simulink library "WECSim_Lib"  (R2019b)
settings: Solver=ode45  StartTime=0.0  StopTime=10.0  RelTol=1e-3  EnableMultiTasking=on
undefined symbols (not defined in the file): body, constraint, mooring, pto, simu, waves, X, Y, Z
libraries: nesl_utility x124, sm_lib x101, $bdroot x14, vrlib x2
(part 1 of 9)
settings Model: Creator=cmichel  LastModifiedBy=ntom
settings DataIOCC: LimitDataPoints=on  SaveFormat=Array  SignalLoggingSaveFormat=ModelDataLogs  ReturnWorkspaceOutputs=off
settings OptimizationCC: LifeSpan=inf
settings DebuggingCC: UnderspecifiedInitializationDetection=Classic  MergeDetectMultiDrivingBlocksExec=none  SolverPrmCheckMsg=warning  MultiTaskDSMMsg=warning  MultiTaskCondExecSysMsg=none  AllowSymbolicDim=off  SFUnexpectedBacktrackingDiag=warning  SFNoUnconditionalDefaultTransitionDiag=warning  SFExecutionAtInitializationDiag=none  ArithmeticOperatorsInVariantConditions=warning
settings HardwareCC: ProdBitPerPointer=32  ProdBitPerSizeT=32  ProdBitPerPtrDiffT=32  ProdLargestAtomicFloat=None  ProdIntDivRoundTo=Undefined  ProdEndianess=Unspecified  ProdWordSize=32  ProdHWDeviceType=32-bit Generic
settings ModelReferenceCC: PropagateSignalLabelsOutOfModel=off
settings SFSimCC: SimUseLocalCustomCode=off  CustomCodeUndefinedFunction=UseInterfaceOnly
settings RTWCC: RTWUseLocalCustomCode=off
settings CodeAppCC: StateflowObjectComments=on
settings GRTTargetCC: TargetLangStandard=C89/C90 (ANSI)
settings ConfigComp: CovMetricSettings=dw  CovSaveCumulativeToWorkspaceVar=on  CovSaveSingleToWorkspaceVar=on  CovExternalEMLEnable=off  CovSFcnEnable=off

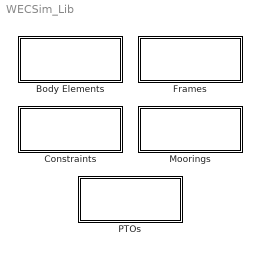
== system WECSim_Lib ==
  Body Elements : Subsystem
      mask Display: text(0,0,' ')
  Constraints : Subsystem
      mask Display: text(0,0,' ')
  Frames : Subsystem
      mask Display: text(0,0,' ')
  Moorings : Subsystem
      mask Display: text(0,0,' ')
  PTOs : Subsystem
      mask Display: text(0,0,' ')

== system WECSim_Lib/Body Elements ==
  Flex Body : Subsystem  VariantControl=(default)  mask(Flex Body){body=body(1), InputFileText=Global Reference Frame option "Use Input File" is selected., h5File=hydroData/*.h5, geometryFile=geometry/*.stl, mass=0, momOfInertia=0 0 0, nhBody=0, flexHydroBody=1, cg=0 0 0, cb=0 0 0, dof=, dispVol=0, initLinDisp=0 0 0, initAngularDispAxis=0 1 0, initAngularDispAngle=0, cd=0 0 0, ca=0 0 0, characteristicArea=0 0 0, VME=0, rgME=0 0 0, z=0 0 1}
      mask prompts: body "Body Number:"; mass "Body Mass [kg]:"; momOfInertia "MoI [kg*m^2]:"; nhBody "Non-hydro Body"; flexHydroBody "Flexible Body"; cg "Center of gravity [m]"; cb "Center of buoyancy [m]"; dof "Degrees of freedom"; dispVol "Displaced Volume [m^3]"; initLinDisp "Initial Linear Displacement"; initAngularDispAxis "Initial Angular Displacement Axis"; initAngularDispAngle "Initial Angular Displacement"; cd "Drag coefficient"; ca "Added mass coefficient"; characteristicArea "Characteristic Area"; VME "Characteristic Volume"; rgME "Point of Application"; z "Z axis"
      mask help:
      | A Flex Body may contain generalized body modes that account for various bending, shear or other deformation modes. The BEM output must contain data for these additional DOFs.
      |
      | The variable name input below must be 'body(i)' where i=1,2,...
      | body(i) must be defined in the input file with the following fields:
      |
      |     .flexHydroBody = 1 (required)
      |             Float.
      |             Flag that creates a flex body. Set equal to 1 if the BEM data contains more than 6 degrees of freedom.
      |     .filename (required)
      |             String.
      |             The file path specifying the .h5 file for the body.
      |     .mass (required)
      |             Float or string.
      |             The translational interia or mass of the body in kg. If a string, the value must be 'equilibrium'. Default = [ ]
      |     .momOfIntertia (required)
      |             3x1 vector [Ixx Iyy Izz].
      |             Rotational intertia of the body in kg*m^2. Default = [ ]
      |     .geometryFile (optional)
      |             String
      |             Path to the geometry file of the body (.stl). Required for nonlinear hydrodynamics or visualization. Default = [ ]
      mask init:
      | if exist('body','var')
      |     % geometry file name
      |     h=[gcb '/Structure/Body Properties'];
      |     geomFile=body.geometryFile;
      |     set_param(h,'ExtGeomFileName',geomFile);
      |     geomType='STL';
      |     % split version e.g. '9.10.0.16028 (R2021a)' into 9, 10, 0, NaN.
      |     % cannot compare str2double('9.10') because it becomes '9.1' 
      |     ver=split(version,'.');
      |     ver=str2double(ver(1:3));
      |     if ver(1) < 9 || (ver(1) == 9 && ver(2) < 6)
      |        set_param(h,'ExtGeomFileType',geomType);
      |     end
      |     % toWorkSpace: outputs
      |     h=[gcb '/To Workspace'];
      |     responseName=['body' num2str(body.bodyNumber) '_out'];
      |     set_param(h,'VariableName',responseName);
      |     % toWorkSpace: hydrostatic pressures
      |     h=[gcb '/Hydrostatic Restoring Force Calculation/Hydrostatic Restoring Force Calculation/Linear and Nonlinear Restoring Force Variant Subsystem/Nonlinear Hydrostatic Restoring Force/To Workspace1'];
      |     responseName=['body' num2str(body.bodyNumber) '_hspressure_out'];
      |     set_param(h,'VariableName',responseName); 
      |     % toWorkSpace: wave pressures (non-linear Freude-Krylov)
      |     h=[gcb '/Wave Diffraction and Excitation Force Calculation/Wave Diffraction and Excitation Force Calculation/Nonlinear FK Force Variant Subsystem/With Nonlinear FroudeKrylov Force/To Workspace'];
      |     responseName=['body' num2str(body.bodyNumber) '_wavenonlinearpressure_out'];
      |     set_param(h,'VariableName',responseName);
      |     % toWorkSpace: wave pressures (linear Freude-Krylov)
      |     h=[gcb '/Wave Diffraction and Excitation Force Calculation/Wave Diffraction and Excitation Force Calculation/Nonlinear FK Force Variant Subsystem/With Nonlinear FroudeKrylov Force/To Workspace1'];
      |     responseName=['body' num2str(body.bodyNumber) '_wavelinearpressure_out'];
      |     set_param(h,'VariableName',responseName);
      |     % position GoTo 
      |     h=[gcb '/Goto'];
      |     responseName=['disp' num2str(body.bodyNumber)];
      |     set_param(h,'GotoTag',responseName);
      |     % position From
      |     h=[gcb '/From'];
      |     responseName=['disp' num2str(body.bodyNumber)];
      |     set_param(h,'GotoTag',responseName);
      |     % velocity GoTo 
      |     h=[gcb '/Goto1'];
      |     responseName=['vel' num2str(body.bodyNumber)];
      |     set_param(h,'GotoTag',responseName);
      |     % velocity From 
      |     h=[gcb '/From1'];
      |     responseName=['vel' num2str(body.bodyNumber)];
      |     set_param(h,'GotoTag',responseName);
      |     % acceleration GoTo 
      |     h=[gcb '/Goto2'];
      |     responseName=['acc' num2str(body.bodyNumber)];
      |     set_param(h,'GotoTag',responseName);
      |     % acceleration From 
      |     h=[gcb '/From2'];
      |     responseName=['acc' num2str(body.bodyNumber)];
      |     set_param(h,'GotoTag',responseName);
      | end
      mask Help:
      | A Flex Body may contain generalized body modes that account for various bending, shear or other deformation modes. The BEM output must contain data for these additional DOFs.
      | 
      | The variable name input below must be 'body(i)' where i=1,2,...
      | body(i) must be defined in the input file with the following fields:
      | 
      |     .flexHydroBody = 1 (required)
      |             Float.
      |             Flag that creates a flex body. Set equal to 1 if the BEM data contains more than 6 degrees of freedom.
      |     .filename (required)
      |             String.
      |             The file path specifying the .h5 file for the body.
      |     .mass (required)
      |             Float or string.
      |             The translational interia or mass of the body in kg. If a string, the value must be 'equilibrium'. Default = [ ]
      |     .momOfIntertia (required)
      |             3x1 vector [Ixx Iyy Izz].
      |             Rotational intertia of the body in kg*m^2. Default = [ ]
      |     .geometryFile (optional)
      |             String
      |             Path to the geometry file of the body (.stl). Required for nonlinear hydrodynamics or visualization. Default = [ ]
      mask TypeOptions nhBody: 0 | 1 | 2
      mask Callback nhBody: bodyClassCallback(gcbh)
      mask TypeOptions flexHydroBody: 0 | 1
      mask DialogControl ParameterGroupVar Prompt: Custom Parameters
      mask DialogControl std_opts Prompt: Standard Options
      mask DialogControl H5button Prompt: Select .h5 File
      mask DialogControl H5button Callback: h5ButtonCallback(gcbh)
      mask DialogControl STLbutton Prompt: Select .stl File
      mask DialogControl STLbutton Callback: stlButtonCallback(gcbh)
      mask DialogControl momOfInertia Tooltip: Moment of Inertia
      mask DialogControl initDisp Prompt: Initial Displacement
      mask DialogControl morisonElement Prompt: Morison Element
      mask DialogControl rgME Tooltip: The vector from the body COG to point of application for the Morison Element
      mask DialogControl z Tooltip: The unit normal vector center axis of the Morison Element
  Rigid Body : Subsystem  Variant=on  AllowZeroVariantControls=on  mask(Rigid Body){body=body(1), InputFileText=Global Reference Frame option "Use Input File" is selected., h5File=hydroData/*.h5, geometryFile=geometry/*.stl, mass=0, momOfInertia=0 0 0, nhBody=0, flexHydroBody=0, cg=0 0 0, cb=0 0 0, dof=6, dispVol=0, initLinDisp=0 0 0, initAngularDispAxis=0 1 0, initAngularDispAngle=0, cd=0 0 0, ca=0 0 0, characteristicArea=0 0 0, VME=0, rgME=0 0 0, z=0 0 1}
      mask prompts: body "Body Number:"; mass "Body Mass [kg]:"; momOfInertia "MoI [kg*m^2]:"; nhBody "Non-hydro Body"; flexHydroBody "Flexible Body"; cg "Center of gravity [m]"; cb "Center of buoyancy [m]"; dof "Degrees of freedom"; dispVol "Displaced Volume [m^3]"; initLinDisp "Initial Linear Displacement"; initAngularDispAxis "Initial Angular Displacement Axis"; initAngularDispAngle "Initial Angular Displacement"; cd "Drag coefficient"; ca "Added mass coefficient"; characteristicArea "Characteristic Area"; VME "Characteristic Volume"; rgME "Point of Application"; z "Z axis"
      mask help:
      | A rigid body has no generalized body modes. It can be a standard hydrodynamic body, a drag body, or a non-hydrodynamic body.
      |
      | The variable name input below must be 'body(i)' where i=1,2,...
      | body(i) must be defined in the input file with the fields appropriate to each variant.
      mask init:
      | if exist('body','var')
      |     % Hydro Body
      |     h = [gcb '/Hydrodynamic Body'];
      |     responseName = ['sv_b' num2str(body.bodyNumber) '_hydroBody'];
      |     set_param(h,'VariantControl',responseName);
      |     % Hydro Body Morison Element Off
      |     h = [gcb '/Hydrodynamic Body/Morison Element and ViscousDampingForceCalculation/Morison Element Variant Subsystem/Morison Element Off'];
      |     responseName = ['sv_b' num2str(body.bodyNumber) '_MEOff'];
      |     set_param(h,'VariantControl',responseName);
      |     % Hydro Body Morison Element On
      |     h = [gcb '/Hydrodynamic Body/Morison Element and ViscousDampingForceCalculation/Morison Element Variant Subsystem/Morison Element On'];
      |     responseName = ['sv_b' num2str(body.bodyNumber) '_MEOn'];
      |     set_param(h,'VariantControl',responseName);
      |     % Non-Hydro Body
      |     h = [gcb '/Non-Hydro Body'];
      |     responseName = ['sv_b' num2str(body.bodyNumber) '_nonHydroBody'];
      |     set_param(h,'VariantControl',responseName);
      |     % Drag Body
      |     h = [gcb '/Drag Body'];
      |     responseName = ['sv_b' num2str(body.bodyNumber) '_dragBody'];
      |     set_param(h,'VariantControl',responseName);
      |     % Drag Body Morison Element Off
      |     h = [gcb '/Drag Body/Morison Element and ViscousDampingForceCalculation/Morison Element Variant Subsystem/Morison Element Off'];
      |     responseName = ['sv_b' num2str(body.bodyNumber) '_MEOff'];
      |     set_param(h,'VariantControl',responseName);
      |     % Drag Body Morison Element On
      |     h = [gcb '/Drag Body/Morison Element and ViscousDampingForceCalculation/Morison Element Variant Subsystem/Morison Element On'];
      |     responseName = ['sv_b' num2str(body.bodyNumber) '_MEOn'];
      |     set_param(h,'VariantControl',responseName);
      |     % Set zero active variant controls to prevent label issue (works 2017b+)
      |     set_param(gcb,'AllowZeroVariantControls','on');
      | end
      | clear bc h geomFile responseName
      settings: AttributesFormatString=%<body>
      mask Help:
      | A rigid body has no generalized body modes. It can be a standard hydrodynamic body, a drag body, or a non-hydrodynamic body.
      | 
      | The variable name input below must be 'body(i)' where i=1,2,...
      | body(i) must be defined in the input file with the fields appropriate to each variant.
      mask TypeOptions nhBody: 0 | 1 | 2
      mask Callback nhBody: bodyClassCallback(gcbh)
      mask TypeOptions flexHydroBody: 0 | 1
      mask DialogControl ParameterGroupVar Prompt: Custom Parameters
      mask DialogControl H5button Prompt: Select .h5 File
      mask DialogControl H5button Callback: h5ButtonCallback(gcbh)
      mask DialogControl std_opts Prompt: Standard Options
      mask DialogControl STLbutton Prompt: Select .stl File
      mask DialogControl STLbutton Callback: stlButtonCallback(gcbh)
      mask DialogControl momOfInertia Tooltip: Moment of Inertia
      mask DialogControl initDisp Prompt: Initial Displacement
      mask DialogControl morisonElement Prompt: Morison Element
      mask DialogControl rgME Tooltip: The vector from the body COG to point of application for the Morison Element
      mask DialogControl z Tooltip: The unit normal vector center axis of the Morison Element

== system WECSim_Lib/Constraints ==
  Fixed : Subsystem  mask(Constraints){constraint=constraint(1), InputFileText=Global Reference Frame option "Use Input File" is selected., loc=0  0  0, initLinDisp=0 0 0, x=, y=0 1 0, z=0 0 1, upperLimitSpecify=off, upperLimitBound=0, upperLimitTransitionRegionWidth=0, upperLimitStiffness=0, upperLimitDamping=0, lowerLimitSpecify=off, lowerLimitBound=0, lowerLimitTransitionRegionWidth=0, lowerLimitStiffness=0, lowerLimitDamping=0}
      mask prompts: constraint "Constraint Name:"; loc "Location [m]:"; initLinDisp "Initial linear displacement [m]:"; x "X-axis [m]:"; y "Y-axis [m]:"; z "Z-axis [m]:"; upperLimitSpecify "Upper limit"; upperLimitBound "Upper limit bound [m, deg]"; upperLimitTransitionRegionWidth "Upper limit transition region width [m, deg]:"; upperLimitStiffness "Upper limit stiffness [N/m, Nm/rad]:"; upperLimitDamping "Upper limit damping [N/(m/s), Nm/(rad/s)]:"; lowerLimitSpecify "Lower limit"; lowerLimitBound "Upper limit bound [m, deg]:"; lowerLimitTransitionRegionWidth "Upper limit transition region width [m, deg]:"; lowerLimitStiffness "Upper limit stiffness [N/m, Nm/rad]:"; lowerLimitDamping "Upper limit damping [N/(m/s), Nm/(rad/s)]:"
      mask help:
      | Constrains the follower to be fixed relative to the base.
      |
      | The variable name input below must be 'constraint(i)' where i=1,2,...
      | constraint(i) must be defined in the input file with the following fields:
      |
      |     .name (required)
      |             String.
      |             Constraint name. Must comply with Matlab's variable naming rules.
      |     .loc (optional)
      |             3x1 vector [x y z] in meters.
      |             Constraint location. Default = [0 0 0]
      mask init:
      | if exist('constraint','var')
      |     h=[gcb '/output'];
      |     responseName=['constraint' num2str(constraint.constraintNum) '_out'];
      |     set_param(h,'VariableName',responseName);
      | end
      | 
      | constraint.checkLoc('W');
      settings: AttributesFormatString=%<constraint>
      mask Help:
      | Constrains the follower to be fixed relative to the base.
      | 
      | The variable name input below must be 'constraint(i)' where i=1,2,...
      | constraint(i) must be defined in the input file with the following fields:
      | 
      |     .name (required)
      |             String.
      |             Constraint name. Must comply with Matlab's variable naming rules.
      |     .loc (optional)
      |             3x1 vector [x y z] in meters.
      |             Constraint location. Default = [0 0 0]
      mask Callback upperLimitSpecify: hardStopCallback(gcbh)
      mask Callback lowerLimitSpecify: hardStopCallback(gcbh)
      mask DialogControl CusInFile Prompt: Input File
      mask DialogControl ParameterGroupVar Prompt: Custom Parameters
      mask DialogControl std_opts Prompt: Standard options
      mask DialogControl orientations Prompt: Orientation
      mask DialogControl x Tooltip: This axis is defined by the y and z axes.
      mask DialogControl Container7 Prompt: Hard stop
  Floating (3DOF) : Subsystem  mask(Constraints){constraint=constraint(1), InputFileText=Global Reference Frame option "Use Input File" is selected., loc=0  0  0, initLinDisp=0 0 0, x=, y=0 1 0, z=0 0 1, upperLimitSpecify=off, upperLimitBound=0, upperLimitTransitionRegionWidth=0, upperLimitStiffness=0, upperLimitDamping=0, lowerLimitSpecify=off, lowerLimitBound=0, lowerLimitTransitionRegionWidth=0, lowerLimitStiffness=0, lowerLimitDamping=0}
      mask prompts: constraint "Constraint Name:"; loc "Location [m]:"; initLinDisp "Initial linear displacement [m]:"; x "X-axis [m]:"; y "Y-axis [m]:"; z "Z-axis [m]:"; upperLimitSpecify "Upper limit"; upperLimitBound "Upper limit bound [m, deg]"; upperLimitTransitionRegionWidth "Upper limit transition region width [m, deg]:"; upperLimitStiffness "Upper limit stiffness [N/m, Nm/rad]:"; upperLimitDamping "Upper limit damping [N/(m/s), Nm/(rad/s)]:"; lowerLimitSpecify "Lower limit"; lowerLimitBound "Upper limit bound [m, deg]:"; lowerLimitTransitionRegionWidth "Upper limit transition region width [m, deg]:"; lowerLimitStiffness "Upper limit stiffness [N/m, Nm/rad]:"; lowerLimitDamping "Upper limit damping [N/(m/s), Nm/(rad/s)]:"
      mask help:
      | Constraints the follower to planar motion relative to the base, linear
      | motions in the constraint's X- and Z- directions and rotational motion
      | about the constraint's Y-axis.
      |
      |
      | The variable name input below must be 'constraint(i)' where i=1,2,...
      | constraint(i) must be defined in the input file with the following fields:
      |
      |     .name (required)
      |             String.
      |             Constraint name. Must comply with Matlab's variable naming rules.
      |     .loc (optional)
      |             3x1 vector [x y z] in meters.
      |             Constraint location. Default = [0 0 0]
      |     .orientation.z (optional)
      |             3x1 vector [x y z].
      |             Direction of the constraint's Z-coordinate. Default = [0 0 1]
      |     .orientation.y (optional)
      |             3x1 vector [x y z].
      |             Direction of the constraint's Y-coordinate. Default = [0 1 0]
      mask init: same as WECSim_Lib/Constraints/Fixed
      settings: AttributesFormatString=%<constraint>
      mask Help:
      | Constraints the follower to planar motion relative to the base, linear
      | motions in the constraint's X- and Z- directions and rotational motion
      | about the constraint's Y-axis.
      | 
      | 
      | The variable name input below must be 'constraint(i)' where i=1,2,...
      | constraint(i) must be defined in the input file with the following fields:
      | 
      |     .name (required)
      |             String.
      |             Constraint name. Must comply with Matlab's variable naming rules.
      |     .loc (optional)
      |             3x1 vector [x y z] in meters.
      |             Constraint location. Default = [0 0 0]
      |     .orientation.z (optional)
      |             3x1 vector [x y z].
      |             Direction of the constraint's Z-coordinate. Default = [0 0 1]
      |     .orientation.y (optional)
      |             3x1 vector [x y z].
      |             Direction of the constraint's Y-coordinate. Default = [0 1 0]
      mask Callback upperLimitSpecify: hardStopCallback(gcbh)
      mask Callback lowerLimitSpecify: hardStopCallback(gcbh)
      mask DialogControl CusInFile Prompt: Input File
      mask DialogControl ParameterGroupVar Prompt: Custom Parameters
      mask DialogControl std_opts Prompt: Standard options
      mask DialogControl orientations Prompt: Orientation
      mask DialogControl x Tooltip: This axis is defined by the y and z axes.
      mask DialogControl Container7 Prompt: Hard stop
  Floating (6DOF) : Subsystem  mask(Constraints){constraint=constraint(1), InputFileText=Global Reference Frame option "Use Input File" is selected., loc=0  0  0, initLinDisp=0 0 0, x=, y=0 1 0, z=0 0 1, upperLimitSpecify=off, upperLimitBound=0, upperLimitTransitionRegionWidth=0, upperLimitStiffness=0, upperLimitDamping=0, lowerLimitSpecify=off, lowerLimitBound=0, lowerLimitTransitionRegionWidth=0, lowerLimitStiffness=0, lowerLimitDamping=0}
      mask prompts: constraint "Constraint Name:"; loc "Location [m]:"; initLinDisp "Initial linear displacement [m]:"; x "X-axis [m]:"; y "Y-axis [m]:"; z "Z-axis [m]:"; upperLimitSpecify "Upper limit"; upperLimitBound "Upper limit bound [m, deg]"; upperLimitTransitionRegionWidth "Upper limit transition region width [m, deg]:"; upperLimitStiffness "Upper limit stiffness [N/m, Nm/rad]:"; upperLimitDamping "Upper limit damping [N/(m/s), Nm/(rad/s)]:"; lowerLimitSpecify "Lower limit"; lowerLimitBound "Upper limit bound [m, deg]:"; lowerLimitTransitionRegionWidth "Upper limit transition region width [m, deg]:"; lowerLimitStiffness "Upper limit stiffness [N/m, Nm/rad]:"; lowerLimitDamping "Upper limit damping [N/(m/s), Nm/(rad/s)]:"
      mask help:
      | Allows unconstrained motion of the follower relative to the base in all 6
      | degrees of freedom.
      |
      |
      | The variable name input below must be 'constraint(i)' where i=1,2,...
      | constraint(i) must be defined in the input file with the following fields:
      |
      |     .name (required)
      |             String.
      |             Constraint name. Must comply with Matlab's variable naming rules.
      |     .loc (optional)
      |             3x1 vector [x y z] in meters.
      |             Constraint location. Default = [0 0 0]
      |     .orientation.z (optional)
      |             3x1 vector [x y z].
      |             Direction of the constraint's Z-coordinate. Default = [0 0 1]
      |     .orientation.y (optional)
      |             3x1 vector [x y z].
      |             Direction of the constraint's Y-coordinate. Default = [0 1 0]
      mask init: same as WECSim_Lib/Constraints/Fixed
      settings: AttributesFormatString=%<constraint>
      mask Help:
      | Allows unconstrained motion of the follower relative to the base in all 6
      | degrees of freedom.
      | 
      | 
      | The variable name input below must be 'constraint(i)' where i=1,2,...
      | constraint(i) must be defined in the input file with the following fields:
      | 
      |     .name (required)
      |             String.
      |             Constraint name. Must comply with Matlab's variable naming rules.
      |     .loc (optional)
      |             3x1 vector [x y z] in meters.
      |             Constraint location. Default = [0 0 0]
      |     .orientation.z (optional)
      |             3x1 vector [x y z].
      |             Direction of the constraint's Z-coordinate. Default = [0 0 1]
      |     .orientation.y (optional)
      |             3x1 vector [x y z].
      |             Direction of the constraint's Y-coordinate. Default = [0 1 0]
      mask Callback upperLimitSpecify: hardStopCallback(gcbh)
      mask Callback lowerLimitSpecify: hardStopCallback(gcbh)
      mask DialogControl CusInFile Prompt: Input File
      mask DialogControl ParameterGroupVar Prompt: Custom Parameters
      mask DialogControl std_opts Prompt: Standard options
      mask DialogControl orientations Prompt: Orientation
      mask DialogControl x Tooltip: This axis is defined by the y and z axes.
      mask DialogControl Container7 Prompt: Hard stop
  Rotational : Subsystem  mask(Constraints){constraint=constraint(1), InputFileText=Global Reference Frame option "Use Input File" is selected., loc=0  0  0, initLinDisp=0 0 0, x=, y=0 1 0, z=0 0 1, upperLimitSpecify=off, upperLimitBound=0, upperLimitTransitionRegionWidth=0, upperLimitStiffness=0, upperLimitDamping=0, lowerLimitSpecify=off, lowerLimitBound=0, lowerLimitTransitionRegionWidth=0, lowerLimitStiffness=0, lowerLimitDamping=0}
      mask prompts: constraint "Constraint Name:"; loc "Location [m]:"; initLinDisp "Initial linear displacement [m]:"; x "X-axis [m]:"; y "Y-axis [m]:"; z "Z-axis [m]:"; upperLimitSpecify "Upper limit"; upperLimitBound "Upper limit bound [m, deg]"; upperLimitTransitionRegionWidth "Upper limit transition region width [m, deg]:"; upperLimitStiffness "Upper limit stiffness [N/m, Nm/rad]:"; upperLimitDamping "Upper limit damping [N/(m/s), Nm/(rad/s)]:"; lowerLimitSpecify "Lower limit"; lowerLimitBound "Upper limit bound [m, deg]:"; lowerLimitTransitionRegionWidth "Upper limit transition region width [m, deg]:"; lowerLimitStiffness "Upper limit stiffness [N/m, Nm/rad]:"; lowerLimitDamping "Upper limit damping [N/(m/s), Nm/(rad/s)]:"
      mask help:
      | Constraints the follower to rotational motion relative to the base, about
      | the constraint's Y-axis. Location is required and affects dynamics.
      |
      |
      | The variable name input below must be 'constraint(i)' where i=1,2,...
      | constraint(i) must be defined in the input file with the following fields:
      |
      |     .name (required)
      |             String.
      |             Constraint name. Must comply with Matlab's variable naming rules.
      |     .loc (required)
      |             3x1 vector [x y z] in meters.
      |             Constraint location. Default = [0 0 0]
      |     .orientation.z (optional)
      |             3x1 vector [x y z].
      |             Direction of the constraint's Z-coordinate. Default = [0 0 1]
      |     .orientation.y (optional)
      |             3x1 vector [x y z].
      |             Direction of the constraint's Y-coordinate. Default = [0 1 0]
      mask init:
      | if exist('constraint','var')
      |     h=[gcb '/output'];
      |     responseName=['constraint' num2str(constraint.constraintNum) '_out'];
      |     set_param(h,'VariableName',responseName);
      |      h=[gcb '/CONSTRAINT (Revolute Joint)'];
      |     try % this should catch any version issue for which these parameters do not exist
      |         set_param(h,'upperLimitSpecify',constraint.hardStops.upperLimitSpecify)
      |         set_param(h,'lowerLimitSpecify',constraint.hardStops.lowerLimitSpecify)
      |     end
      | end
      | 
      | constraint.checkLoc('E');
      settings: AttributesFormatString=%<constraint>
      mask Help:
      | Constraints the follower to rotational motion relative to the base, about
      | the constraint's Y-axis. Location is required and affects dynamics.
      | 
      | 
      | The variable name input below must be 'constraint(i)' where i=1,2,...
      | constraint(i) must be defined in the input file with the following fields:
      | 
      |     .name (required)
      |             String.
      |             Constraint name. Must comply with Matlab's variable naming rules.
      |     .loc (required)
      |             3x1 vector [x y z] in meters.
      |             Constraint location. Default = [0 0 0]
      |     .orientation.z (optional)
      |             3x1 vector [x y z].
      |             Direction of the constraint's Z-coordinate. Default = [0 0 1]
      |     .orientation.y (optional)
      |             3x1 vector [x y z].
      |             Direction of the constraint's Y-coordinate. Default = [0 1 0]
      mask Callback upperLimitSpecify: hardStopCallback(gcbh)
      mask Callback lowerLimitSpecify: hardStopCallback(gcbh)
      mask DialogControl CusInFile Prompt: Input File
      mask DialogControl ParameterGroupVar Prompt: Custom Parameters
      mask DialogControl std_opts Prompt: Standard options
      mask DialogControl orientations Prompt: Orientation
      mask DialogControl x Tooltip: This axis is defined by the y and z axes.
      mask DialogControl Container7 Prompt: Hard stop
  Translational : Subsystem  mask(Constraints){constraint=constraint(1), InputFileText=Global Reference Frame option "Use Input File" is selected., loc=0  0  0, initLinDisp=0 0 0, x=, y=0 1 0, z=0 0 1, upperLimitSpecify=off, upperLimitBound=0, upperLimitTransitionRegionWidth=0, upperLimitStiffness=0, upperLimitDamping=0, lowerLimitSpecify=off, lowerLimitBound=0, lowerLimitTransitionRegionWidth=0, lowerLimitStiffness=0, lowerLimitDamping=0}
      mask prompts: constraint "Constraint Name:"; loc "Location [m]:"; initLinDisp "Initial linear displacement [m]:"; x "X-axis [m]:"; y "Y-axis [m]:"; z "Z-axis [m]:"; upperLimitSpecify "Upper limit"; upperLimitBound "Upper limit bound [m, deg]"; upperLimitTransitionRegionWidth "Upper limit transition region width [m, deg]:"; upperLimitStiffness "Upper limit stiffness [N/m, Nm/rad]:"; upperLimitDamping "Upper limit damping [N/(m/s), Nm/(rad/s)]:"; lowerLimitSpecify "Lower limit"; lowerLimitBound "Upper limit bound [m, deg]:"; lowerLimitTransitionRegionWidth "Upper limit transition region width [m, deg]:"; lowerLimitStiffness "Upper limit stiffness [N/m, Nm/rad]:"; lowerLimitDamping "Upper limit damping [N/(m/s), Nm/(rad/s)]:"
      mask help:
      | Constraints the follower to translational motion relative to the base, in the constraint's Z-direction.
      |
      |
      | The variable name input below must be 'constraint(i)' where i=1,2,...
      | constraint(i) must be defined in the input file with the following fields:
      |
      |     .name (required)
      |             String.
      |             Constraint name. Must comply with Matlab's variable naming rules.
      |     .loc (optional)
      |             3x1 vector [x y z] in meters.
      |             Constraint location. Default = [0 0 0]
      |     .orientation.z (optional)
      |             3x1 vector [x y z].
      |             Direction of the constraint's Z-coordinate. Default = [0 0 1]
      |     .orientation.y (optional)
      |             3x1 vector [x y z].
      |             Direction of the constraint's Y-coordinate. Default = [0 1 0]
      mask init:
      | if exist('constraint','var')
      |     h=[gcb '/output'];
      |     responseName=['constraint' num2str(constraint.constraintNum) '_out'];
      |     set_param(h,'VariableName',responseName);
      |     h=[gcb '/CONSTRAINT (Prismatic Joint)'];
      |     try % this should catch any version issue for which these parameters do not exist
      |         set_param(h,'upperLimitSpecify',constraint.hardStops.upperLimitSpecify)
      |         set_param(h,'lowerLimitSpecify',constraint.hardStops.lowerLimitSpecify)
      |     end
      | end
      | constraint.checkLoc('W');
      settings: AttributesFormatString=%<constraint>
      mask Help:
      | Constraints the follower to translational motion relative to the base, in the constraint's Z-direction.
      | 
      | 
      | The variable name input below must be 'constraint(i)' where i=1,2,...
      | constraint(i) must be defined in the input file with the following fields:
      | 
      |     .name (required)
      |             String.
      |             Constraint name. Must comply with Matlab's variable naming rules.
      |     .loc (optional)
      |             3x1 vector [x y z] in meters.
      |             Constraint location. Default = [0 0 0]
      |     .orientation.z (optional)
      |             3x1 vector [x y z].
      |             Direction of the constraint's Z-coordinate. Default = [0 0 1]
      |     .orientation.y (optional)
      |             3x1 vector [x y z].
      |             Direction of the constraint's Y-coordinate. Default = [0 1 0]
      mask Callback upperLimitSpecify: hardStopCallback(gcbh)
      mask Callback lowerLimitSpecify: hardStopCallback(gcbh)
      mask DialogControl CusInFile Prompt: Input File
      mask DialogControl ParameterGroupVar Prompt: Custom Parameters
      mask DialogControl std_opts Prompt: Standard options
      mask DialogControl orientations Prompt: Orientation
      mask DialogControl x Tooltip: This axis is defined by the y and z axes.
      mask DialogControl Container7 Prompt: Hard stop

== system WECSim_Lib/Frames ==
  Global Reference Frame : Subsystem  StopFcn=run('wecSimStopFunction')  mask(Frames){waves=waves, simu=simu, ParamInput=Custom Parameters, InputFile=wecSimInputFile.m, mode=normal, explorer=off, solver=ode4, startTime=0, rampTime=100, endTime=400, dt=0.1, CITime=60, ssCalc=0, morisonElement=0, WaveClass=regular, H=2.5, T=8, etaDataFile=NOT DEFINED, spectrumDataFile=NOT DEFINED, waveDir=0, waveSpread=1, spectrumType=NOT DEFINED, freqDisc=EqualEnergy, phaseSeed=0}
      mask prompts: waves "Wave Class Name"; simu "Simulation Class Name"; ParamInput "Parameter Input Method"; mode "Simulation Mode:"; explorer "SimMechanics Explorer:"; solver "SimSolver:"; startTime "Start Time [s]:"; rampTime "Ramp Time [s]:"; endTime "End Time [s]:"; dt "Step Size [s]:"; CITime "CI Time [s]:"; ssCalc "Turn on State Space"; morisonElement "Turn on Morison Element"; WaveClass "Select Wave Class:"; H "Wave Height [m]:"; T "Wave Period [s]:"; waveDir "Wave Direction [deg]:"; waveSpread "Wave Spread [0-1]:"; spectrumType "Wave Spectrum Type:"; freqDisc "Frequency Discretization:"; phaseSeed "Phase Seed:"
      mask help:
      | This block contains Global References, including solver configurations, free surface and seabed description, and simulation time.
      | It uses the following fields from the Simulation and Wave classes:
      |
      | Simulation Class:
      |     .endTime
      |     .dt
      |     .domainSize
      |
      | Wave Class:
      |     .waterDepth
      mask Help:
      | This block contains Global References, including solver configurations, free surface and seabed description, and simulation time.
      | It uses the following fields from the Simulation and Wave classes:
      | 
      | Simulation Class:
      |     .endTime
      |     .dt
      |     .domainSize
      | 
      | Wave Class:
      |     .waterDepth
      mask TypeOptions ParamInput: Input File | Custom Parameters
      mask Callback ParamInput: inputOrCustomCallback(gcbh)
      mask TypeOptions mode: normal | accelerator | rapid-accelerator
      mask TypeOptions explorer: on | off
      mask TypeOptions solver: ode4 | ode45
      mask TypeOptions ssCalc: 0 | 1
      mask TypeOptions morisonElement: 0 | 1
      mask Callback morisonElement: bodyClassCallback(gcbh)
      mask TypeOptions WaveClass: noWaveCIC | regular | regularCIC | irregular | spectrumImport | etaImport
      mask Callback WaveClass: waveClassCallback(gcbh)
      mask TypeOptions spectrumType: PM | JS | NOT DEFINED
      mask TypeOptions freqDisc: EqualEnergy | Traditional
      mask DialogControl CusInFile Prompt: Input File
      mask DialogControl InFileButton Prompt: Select File
      mask DialogControl InFileButton Callback: inFileButtonCallback(gcbh)
      mask DialogControl LoadParam Prompt: Load parameters from Input File
      mask DialogControl LoadParam Callback: loadInputFileCallback(gcbh)
      mask DialogControl ParameterGroupVar Prompt: Custom Parameters
      mask DialogControl SimData Prompt: Simulation Data
      mask DialogControl WaveInfo Prompt: Wave Information
      mask DialogControl ETAbutton Prompt: Select etaData.mat file
      mask DialogControl ETAbutton Callback: etaButtonCallback(gcbh)
      mask DialogControl SpecButton Prompt: Select spectrumData.mat file
      mask DialogControl SpecButton Callback: spectrumButtonCallback(gcbh)
      mask Display: fprintf('Active Method: \n%s',get_param(gcbh,'ParamInput'))

== system WECSim_Lib/Moorings ==
  MoorDyn : Subsystem  mask(MoorDyn){mooring=mooring(1), InputFileText=Global Reference Frame option "Use Input File" is selected., MooringRef=0  0  0, moorDynNodes=0, moorDynLines=0}
      mask prompts: mooring "Mooring Name:"; MooringRef "Reference Location [m]:"; moorDynNodes "Number of MoorDyn Nodes:"; moorDynLines "Number of MoorDyn Lines:"
      mask help:
      | A mooring body that applies stiffness, damping and pretensions forces to the follower using a MoorDyn simulation. The response of the mooring body is relative to the global reference frame.
      |
      | The variable name input below must be 'mooring(i)' where i=1,2,...
      | mooring(i) must be defined in the input file with the following fields:
      |
      |     .name (required)
      |             String.
      |             Mooring name. Must comply with Matlab's variable naming rules.
      |     .ref (optional)
      |             3x1 vector [x y z] in meters.
      |             Mooring location. Default = [0 0 0]
      |     .initDisp (optional)
      |             Struct
      |             Contains the initial position, angle and axis of the mooring body.
      |     .initDisp.initLinDisp (optional)
      |             3x1 vector [x y z] in meters.
      |             Initial linear displacement from the ref position. Default = [0 0 0]
      |             This can can be set directly or with the setInitDisp() method.
      |     .initDisp.initAngularDispAxis (optional)
      |             3x1 vector [x y z]
      |             Initial angular displacement axis. Default = [0 1 0]
      |             This can can be set directly or with the setInitDisp() method.
      |     .initDisp.initAngularDispAngle (optional)
      |             Float.
      |             Initial angular displacement angle about initAngularDispAxis in radians. Default = [0 0 0]
      |             This can can be set directly or with the setInitDisp() method.
      |     .moorDynLines (optional)
      |             Float.
      |             Number of lines for MoorDyn to use. Default = 0
      |     .moorDynNodes (optional)
      |             moorDynLines x 1 vector.
      |             Specifies the number of nodes per line in MoorDyn. Default = []
      mask init:
      | if exist('mooring','var')
      |     % toWorkSpace: outputs
      |     h=[gcb '/To Workspace'];
      |     responseName=['mooring' num2str(mooring.mooringNum) '_out'];
      |     set_param(h,'VariableName',responseName);
      | end
      | 
      | mooring.moorDyn = 1;
      | mooring.moorDynInput();
      settings: AttributesFormatString=%<mooring>
      mask Help:
      | A mooring body that applies stiffness, damping and pretensions forces to the follower using a MoorDyn simulation. The response of the mooring body is relative to the global reference frame.
      | 
      | The variable name input below must be 'mooring(i)' where i=1,2,...
      | mooring(i) must be defined in the input file with the following fields:
      | 
      |     .name (required)
      |             String.
      |             Mooring name. Must comply with Matlab's variable naming rules.
      |     .ref (optional)
      |             3x1 vector [x y z] in meters.
      |             Mooring location. Default = [0 0 0]
      |     .initDisp (optional)
      |             Struct
      |             Contains the initial position, angle and axis of the mooring body.
      |     .initDisp.initLinDisp (optional)
      |             3x1 vector [x y z] in meters.
      |             Initial linear displacement from the ref position. Default = [0 0 0]
      |             This can can be set directly or with the setInitDisp() method.
      |     .initDisp.initAngularDispAxis (optional)
      |             3x1 vector [x y z]
      |             Initial angular displacement axis. Default = [0 1 0]
      |             This can can be set directly or with the setInitDisp() method.
      |     .initDisp.initAngularDispAngle (optional)
      |             Float.
      |             Initial angular displacement angle about initAngularDispAxis in radians. Default = [0 0 0]
      |             This can can be set directly or with the setInitDisp() method.
      |     .moorDynLines (optional)
      |             Float.
      |             Number of lines for MoorDyn to use. Default = 0
      |     .moorDynNodes (optional)
      |             moorDynLines x 1 vector.
      |             Specifies the number of nodes per line in MoorDyn. Default = []
      mask DialogControl CusInFile Prompt: Input File
      mask DialogControl ParameterGroupVar Prompt: Custom Parameters
  MooringMatrix : Subsystem  mask(Mooring Matrix){mooring=mooring(1), InputFileText=Global Reference Frame option "Use Input File" is selected., ref=0 0 0, preTension=[0 0 0 0 0 0], k={ '0', '0', '0', '0', '0', '0'; '0', '0', '0', '0', '0', '0'; '0', '0', '0', '0', '0', '0'; '0', '0', '0', '0', '0', '0'; '0', '0', '0', '0', '0', '0'; '0', '0', '0', '0', '0', '0' }, c={ '0', '0', '0', '0', '0', '0'; '0', '0', '0', '0', '0', '0'; '0', '0', '0', '0', '0', '0'; '0', '0', '0', '0', '0', '0'; '0', '0', '0', '0', '0', '0'; '0', '0', '0', '0', '0', '0' }}
      mask prompts: mooring "Mooring Name:"; ref "Reference Location [m]:"; preTension "Pretension Force [N]:"; k "Stiffness [N/m]:"; c "Damping [N/m^2]:"
      mask help:
      | A mooring body that applies stiffness, damping and pretensions forces to the follower. The response of the mooring body is relative to the global reference frame.
      |
      | The variable name input below must be 'mooring(i)' where i=1,2,...
      | mooring(i) must be defined in the input file with the following fields:
      |
      |     .name (required)
      |             String.
      |             Mooring name. Must comply with Matlab's variable naming rules.
      |     .ref (optional)
      |             3x1 vector [x y z] in meters.
      |             Mooring location. Default = [0 0 0]
      |     .initDisp (optional)
      |             Struct
      |             Contains the initial position, angle and axis of the mooring body.
      |     .initDisp.initLinDisp (optional)
      |             3x1 vector [x y z] in meters.
      |             Initial linear displacement from the ref position. Default = [0 0 0]
      |             This can can be set directly or with the setInitDisp() method.
      |     .initDisp.initAngularDispAxis (optional)
      |             3x1 vector [x y z]
      |             Initial angular displacement axis. Default = [0 1 0]
      |             This can can be set directly or with the setInitDisp() method.
      |     .initDisp.initAngularDispAngle (optional)
      |             Float.
      |             Initial angular displacement angle about initAngularDispAxis in radians. Default = [0 0 0]
      |             This can can be set directly or with the setInitDisp() method.
      |     .matrix (optional)
      |             Struct
      |             Contains the stiffness matrix, damping matrix and pretension of the mooring body.
      |     .matrix.k (optional)
      |             6x6 vector.
      |             Mooring linear spring stiffness. Default = zeros(6)
      |     .matrix.c (optional)
      |             6x6 vector.
      |             Mooring linear damping coefficient. Default = zeros(6)
      |     .matrix.preTension (optional)
      |             6x1 vector.
      |             Mooring preTension force. Default = [0 0 0 0 0 0]
      mask init:
      | if exist('mooring','var')
      |     % toWorkSpace: outputs
      |     h=[gcb '/To Workspace'];
      |     responseName=['mooring' num2str(mooring.mooringNum) '_out'];
      |     set_param(h,'VariableName',responseName);
      | end
      settings: AttributesFormatString=%<mooring>
      mask Help:
      | A mooring body that applies stiffness, damping and pretensions forces to the follower. The response of the mooring body is relative to the global reference frame.
      | 
      | The variable name input below must be 'mooring(i)' where i=1,2,...
      | mooring(i) must be defined in the input file with the following fields:
      | 
      |     .name (required)
      |             String.
      |             Mooring name. Must comply with Matlab's variable naming rules.
      |     .ref (optional)
      |             3x1 vector [x y z] in meters.
      |             Mooring location. Default = [0 0 0]
      |     .initDisp (optional)
      |             Struct
      |             Contains the initial position, angle and axis of the mooring body.
      |     .initDisp.initLinDisp (optional)
      |             3x1 vector [x y z] in meters.
      |             Initial linear displacement from the ref position. Default = [0 0 0]
      |             This can can be set directly or with the setInitDisp() method.
      |     .initDisp.initAngularDispAxis (optional)
      |             3x1 vector [x y z]
      |             Initial angular displacement axis. Default = [0 1 0]
      |             This can can be set directly or with the setInitDisp() method.
      |     .initDisp.initAngularDispAngle (optional)
      |             Float.
      |             Initial angular displacement angle about initAngularDispAxis in radians. Default = [0 0 0]
      |             This can can be set directly or with the setInitDisp() method.
      |     .matrix (optional)
      |             Struct
      |             Contains the stiffness matrix, damping matrix and pretension of the mooring body.
      |     .matrix.k (optional)
      |             6x6 vector.
      |             Mooring linear spring stiffness. Default = zeros(6)
      |     .matrix.c (optional)
      |             6x6 vector.
      |             Mooring linear damping coefficient. Default = zeros(6)
      |     .matrix.preTension (optional)
      |             6x1 vector.
      |             Mooring preTension force. Default = [0 0 0 0 0 0]
      mask DialogControl CusInFile Prompt: Input File
      mask DialogControl ParameterGroupVar Prompt: Custom Parameters
      mask DialogControl matrix Prompt: Additional Parameters
